simulink model "SWTTEO"  (R2020a)
settings: Solver=VariableStepAuto  StartTime=0.0  StopTime=20  RelTol=1e-3
libraries: dspmlti4 x1, dspfdesign x1, dspsigops x1
settings Model: PauseTimes=2  Creator=diflo  LastModifiedBy=diflo

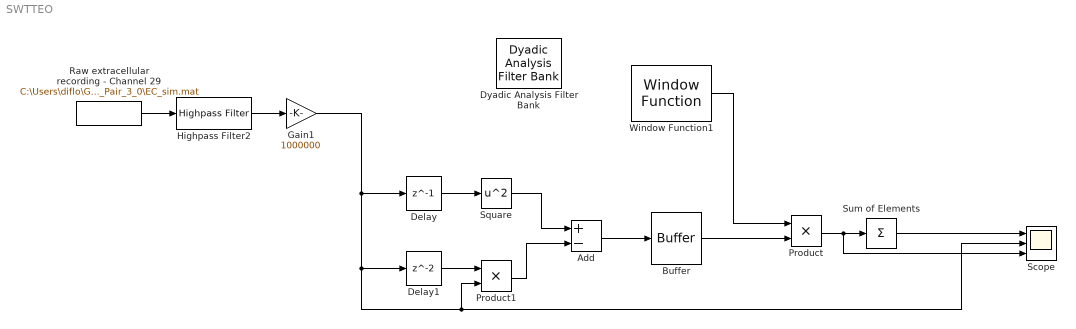
== system SWTTEO ==
  Add : Sum  Inputs=+-
  Buffer : Buffer  N=30  V=29  OutputFrames=off
  Delay : Delay  DelayLength=1  InitialCondition=0  SampleTime=1/30000
  Delay1 : Delay  InitialCondition=0  SampleTime=1/30000
  Dyadic Analysis Filter Bank : dspmlti4/Dyadic Analysis Filter Bank  Wname=User-defined  OrdRec_ordDec=[1 / 1]  Order=2  LPF="[0.0352   -0.0854   -0.1350   0.4599   0.8069   0.3327]"  HPF="[-0.3327    0.8069   -0.4599   -0.1350    0.0854    0.0352]"  NumLevels=2  tree=Asymmetric  Output=Multiple ports  OutputFrames=off
      settings: SourceProductBaseCode=DS
  Gain1 : Gain  Gain=1000000
  Highpass Filter2 : dspfdesign/Highpass Filter  FilterType=IIR  DesignForMinimumOrder=off  FilterOrder=3  StopbandFrequency=1  PassbandFrequency=300  StopbandAttenuation=80  PassbandRipple=0.1  InheritSampleRate=off  SampleRate=30000  SimulateUsing=Interpreted execution  roundingMode=Floor  coeffsDataTypeStr=fixdt(1,16)
  Product : Product
  Product1 : Product
  Raw extracellular recording - Channel 29 : FromFile  FileName=C:\Users\diflo\Google Drive\IIT - Neuroengineering\MathWorks Project\Data\KampffLab\2014_11_25_Pair_3_0\EC_sim.mat  SampleTime=1/30000
  Scope : Scope  NumInputPorts=3
  Square : Math  Operator=square  SaturateOnIntegerOverflow=on
  Sum of Elements : Sum  Inputs=+
  Window Function1 : dspsigops/Window Function  winmode=Generate window  wintype=Hamming  sampmode=Discrete  samptime=1/30000  N=30  Rs=50  beta=10  winsamp=Periodic  UserWindow=hamming  OptParams=off  UserParams={'symmetric'}  dataType=double  isSigned=on  wordLen=16  udDataType=sfix(16)  fracBitsMode=Best precision  numFracBits=15  roundingMode=Floor  overflowMode=off  numSidelobes=4  sidelobeLevel=-30
      settings: SourceProductBaseCode=DS
  wires:
  Raw extracellular recording - Channel 29/1 -> Highpass Filter2/1
  Gain1/1 -> Scope/2, Product1/2, Delay1/1, Delay/1
  Window Function1/1 -> Product/1
  Delay/1 -> Square/1
  Delay1/1 -> Product1/1
  Square/1 -> Add/1
  Product1/1 -> Add/2
  Add/1 -> Buffer/1
  Buffer/1 -> Product/2
  Product/1 -> Scope/3, Sum of Elements/1
  Highpass Filter2/1 -> Gain1/1
  Sum of Elements/1 -> Scope/1
